simulink model "simulink_file_for_r2021b"  (R2021b)
settings: Solver=VariableStepAuto  StartTime=0.0  StopTime=20  RelTol=1e-3
settings Model: Creator=chengouyang  LastModifiedBy=chengouyang
settings DebuggingCC: UnconnectedInputMsg=none  UnconnectedOutputMsg=none  UnconnectedLineMsg=none
settings ModelReferenceCC: EnableRefExpFcnMdlSchedulingChecks=off
settings RTWCC: DLArmComputeVersion=20.02.1

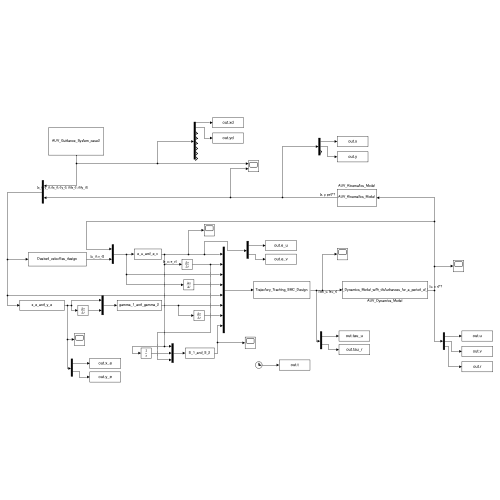
[thumbnail: Simulink's stored preview of the top-level diagram]
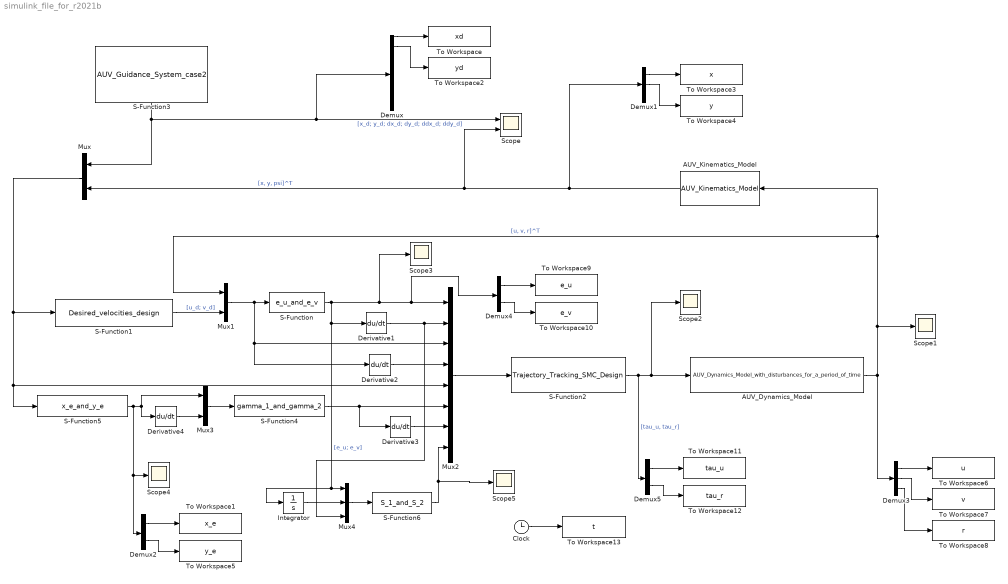
== system simulink_file_for_r2021b ==
  AUV_Dynamics_Model : S-Function  FunctionName=AUV_Dynamics_Model_with_disturbances_for_a_period_of_time  Parameters=pa  SFunctionDeploymentMode=off  EnableBusSupport=off
  AUV_Kinematics_Model : S-Function  FunctionName=AUV_Kinematics_Model  Parameters=pa  SFunctionDeploymentMode=off  EnableBusSupport=off
  Clock : Clock
  Demux : Demux  Outputs=8
  Demux1 : Demux  Outputs=3
  Demux2 : Demux  Outputs=2
  Demux3 : Demux  Outputs=3
  Demux4 : Demux  Outputs=2
  Demux5 : Demux  Outputs=2
  Derivative{1..4} (4 alike) : Derivative
  Integrator : Integrator
  Mux : Mux  Inputs=2
  Mux1 : Mux  Inputs=2
  Mux2 : Mux  Inputs=8
  Mux3 : Mux  Inputs=2
  Mux4 : Mux  Inputs=3
  S-Function : S-Function  FunctionName=e_u_and_e_v  SFunctionDeploymentMode=off  EnableBusSupport=off
  S-Function1 : S-Function  FunctionName=Desired_velocities_design  Parameters=pa  SFunctionDeploymentMode=off  EnableBusSupport=off
  S-Function2 : S-Function  FunctionName=Trajectory_Tracking_SMC_Design  Parameters=pa  SFunctionDeploymentMode=off  EnableBusSupport=off
  S-Function3 : S-Function  FunctionName=AUV_Guidance_System_case2  SFunctionDeploymentMode=off  EnableBusSupport=off
  S-Function4 : S-Function  FunctionName=gamma_1_and_gamma_2  Parameters=pa  SFunctionDeploymentMode=off  EnableBusSupport=off
  S-Function5 : S-Function  FunctionName=x_e_and_y_e  SFunctionDeploymentMode=off  EnableBusSupport=off
  S-Function6 : S-Function  FunctionName=S_1_and_S_2  Parameters=pa  SFunctionDeploymentMode=off  EnableBusSupport=off
  Scope : Scope  NumInputPorts=2
  Scope{1..5} (5 alike) : Scope
  To Workspace : ToWorkspace  VariableName=xd  SampleTime=-1
  To Workspace1 : ToWorkspace  VariableName=x_e  SampleTime=-1
  To Workspace10 : ToWorkspace  VariableName=e_v  SampleTime=-1
  To Workspace11 : ToWorkspace  VariableName=tau_u  SampleTime=-1
  To Workspace12 : ToWorkspace  VariableName=tau_r  SampleTime=-1
  To Workspace13 : ToWorkspace  VariableName=t  SampleTime=-1
  To Workspace2 : ToWorkspace  VariableName=yd  SampleTime=-1
  To Workspace3 : ToWorkspace  VariableName=x  SampleTime=-1
  To Workspace4 : ToWorkspace  VariableName=y  SampleTime=-1
  To Workspace5 : ToWorkspace  VariableName=y_e  SampleTime=-1
  To Workspace6 : ToWorkspace  VariableName=u  SampleTime=-1
  To Workspace7 : ToWorkspace  VariableName=v  SampleTime=-1
  To Workspace8 : ToWorkspace  VariableName=r  SampleTime=-1
  To Workspace9 : ToWorkspace  VariableName=e_u  SampleTime=-1
  wires:
  AUV_Dynamics_Model/1 -> Mux1/1, AUV_Kinematics_Model/1, Scope1/1, Demux3/1  "[u, v, r]^T"
  S-Function2/1 -> Demux5/1, Scope2/1, AUV_Dynamics_Model/1  "[tau_u, tau_r]"
  S-Function3/1 -> Demux/1, Scope/1, Mux/1  "[x_d; y_d; dx_d; dy_d; ddx_d; ddy_d]"
  Mux/1 -> S-Function1/1, S-Function5/1, Mux2/5
  S-Function1/1 -> Mux1/2  "[u_d; v_d]"
  AUV_Kinematics_Model/1 -> Demux1/1, Scope/2, Mux/2  "[x, y, psi]^T"
  Mux1/1 -> Derivative2/1, Mux2/3, S-Function/1
  S-Function/1 -> Scope3/1, Demux4/1, Mux2/1, Derivative1/1, Mux4/1, Integrator/1  "[e_u; e_v]"
  Mux2/1 -> S-Function2/1
  Derivative1/1 -> Mux4/3, Mux2/2
  Derivative2/1 -> Mux2/4
  S-Function4/1 -> Derivative3/1, Mux2/6
  Derivative3/1 -> Mux2/7
  Mux3/1 -> S-Function4/1
  Derivative4/1 -> Mux3/2
  S-Function6/1 -> Scope5/1, Mux2/8
  Integrator/1 -> Mux4/2
  Mux4/1 -> S-Function6/1
  Demux/1 -> To Workspace/1
  Demux/2 -> To Workspace2/1
  Demux1/1 -> To Workspace3/1
  Demux1/2 -> To Workspace4/1
  S-Function5/1 -> Demux2/1, Scope4/1, Derivative4/1, Mux3/1
  Demux2/1 -> To Workspace1/1
  Demux2/2 -> To Workspace5/1
  Demux3/1 -> To Workspace6/1
  Demux3/2 -> To Workspace7/1
  Demux3/3 -> To Workspace8/1
  Demux4/2 -> To Workspace10/1
  Demux4/1 -> To Workspace9/1
  Demux5/2 -> To Workspace12/1
  Demux5/1 -> To Workspace11/1
  Clock/1 -> To Workspace13/1
